simulink model "Combined"  (R2024b)
settings: Solver=VariableStepAuto  StartTime=0.0  StopTime=10.0  RelTol=1e-3
undefined symbols (not defined in the file): C_PFC, Co, Cr, D11, Delta, DiscIntNeverNeededParam, Fnom, Fr_I, fs_LCC_max, fs_LCC_min, Ki_LLC, Ki_V, Kp_I, Kp_LLC, Kp_V, Kr_I, L_PFC, Limit_V, Lm, Lr, Np, Ns, Po_nom, RL_PFC, Ts_Control, Ts_Power, Vnom_ac, Vo_nom, Vref_LCC_max, Vref_LCC_min
libraries: spsSeriesRLCBranchLib x9, spsCurrentMeasurementLib x7, spsDiodeLib x7, MyLibrary x6, spsVoltageMeasurementLib x5, spsMeanLib x4, spsOnDelayLib x3, slpidlib x2, spsPWMGeneratorDCDCLib x2, spsFourierLib x2, simulink x2, spspowerguiLib x2
settings Model: Creator=chang  LastModifiedBy=chang

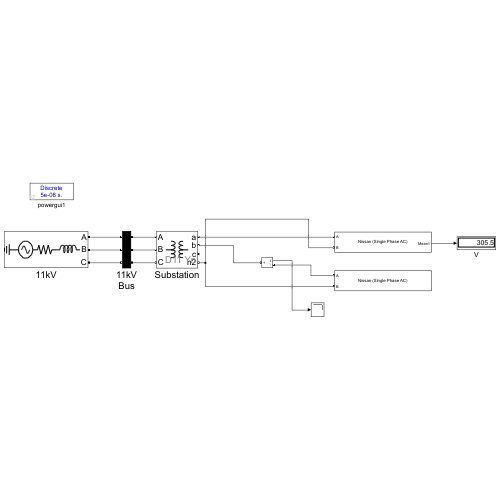
[thumbnail: Simulink's stored preview of the top-level diagram]
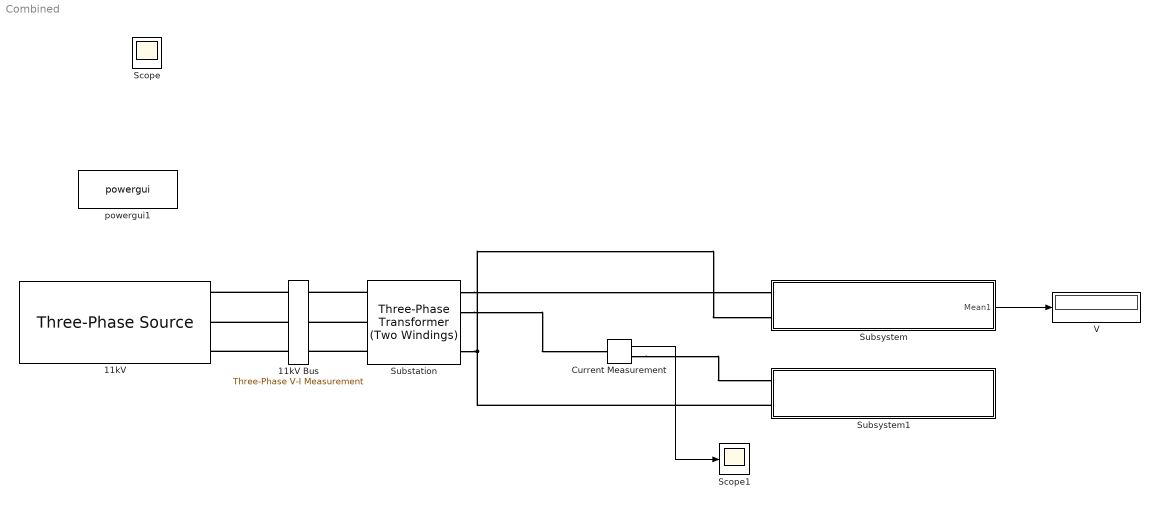
== system Combined ==
  11kV : spsThreePhaseSourceLib/Three-Phase Source  InternalConnection=Yg  VoltagePhases=off  Voltage=11e3  PhaseAngle=0  Voltage_phases=[25e3 25e3 25e3]/sqrt(3)  PhaseAngles_phases=[0 -120 +120]  Frequency=50  NonIdealSource=on  SpecifyImpedance=on  Resistance=0.8929  Inductance=16.58e-3  ShortCircuitLevel=15e6  BaseVoltage=11e3  XRratio=7  BusType=swing  Pref=10e3  Qref=0  Prefabc=[10e3, 10e3, 10e3]  Qrefabc=[0, 0, 0]  Qmin=-inf  Qmax=inf
  11kV Bus : spsThreePhaseVIMeasurementLib/Three-Phase V-I Measurement  VoltageMeasurement=no  SetLabelV=off  LabelV=Vabc  Vpu=off  VpuLL=off  CurrentMeasurement=no  SetLabelI=off  LabelI=Iabc  Ipu=off  Pbase=100e6  Vbase=500e3  OutputType=Complex  PhasorSimulation=off  PSBequivalent=0
  Current Measurement : spsCurrentMeasurementLib/Current Measurement  PhasorSimulation=off  OutputType=Complex  PSBequivalent=0
  Scope1 : Scope
  Substation : spsThreePhaseTransformerTwoWindingsLib/Three-Phase Transformer (Two Windings)  Winding1Connection=Delta (D11)  Winding2Connection=Yn  CoreType=Three single-phase transformers  SetSaturation=off  Hysteresis=off  DataFile='hysteresis'  SetInitialFlux=off  Measurements=None  UNITS=pu  NominalPower=[ 1e6 , 50 ]  Winding1=[11e3 0.0019999 0.080002]  Winding2=[0.4e3 0.002 0.08]  Rm=500.01  Lm=500  L0=0.5  Saturation=[0 0;0.0024 1.2;0.99999 1.52]  InitialFluxes=[ 0.8 , -0.8 , 0.7 ]  BreakLoop=off  DiscreteSolver=Trapezoidal iterative  DataType=off  TransfoNumber=1
  Subsystem : Subsystem
      mask Display: disp('Nissan (Single Phase AC)');
  Subsystem1 : Subsystem
      mask Display: disp('Nissan (Single Phase AC)');
  V : Display
  powergui1 : spspowerguiLib/powergui  Priority=1  SimulationMode=Discrete  SampleTime=Ts_Power  frequency=60  Iterations=50  frequencyindice=0  Pbase=100e6  ErrMax=1e-4  UnitsV=kV  UnitsW=MW  buscounter=0  FunctionMessages=off  echomessages=off  EnableUseOfTLC=off  CurrentSourceSwitches=off  DisableSnubberDevices=off  DisableRonSwitches=off  DisableVfSwitches=off  DisplayEquations=off  AutomaticDiscreteSolvers=off  SolverType=Tustin/Backward Euler (TBE)  Interpol=off  ExternalGateDelay=off  methode=off  Ts=100  x0status=blocks  SPID=on  SwTol=0  HookPort=off  NonlinearTolerance=1e-4  nMaxIteration=100  ContinueOnMaxIteration=off  RestoreLinks=warning  ResistiveCurrentMeasurement=off  Frange=[0:2:500]  Ylog=off  Xlog=on  ShowGrid=off  save=off  variable=ZData  structure=0  ZoomFFT=off  StartTime=0.0  cycles=1  DisplayStyle=1  fundamental=60  FreqAxis=off  MaxFrequency=1000  frequencyindicesteady=1  RmsSteady=1  display=off
  Scope : Scope
  wires:
  Subsystem/1(Mean1) -> V/1
  Current Measurement/1 -> Scope1/1
  connections:
  11kV Bus/LConn1 -- 11kV/RConn1
  11kV Bus/LConn2 -- 11kV/RConn2
  11kV Bus/LConn3 -- 11kV/RConn3
  Substation/LConn1 -- 11kV Bus/RConn1
  Substation/LConn2 -- 11kV Bus/RConn2
  Substation/LConn3 -- 11kV Bus/RConn3
  Substation/RConn4 -- Subsystem1/LConn2 -- Subsystem/LConn2
  Substation/RConn1 -- Subsystem/LConn1
  Current Measurement/RConn1 -- Subsystem1/LConn1
  Substation/RConn2 -- Current Measurement/LConn1

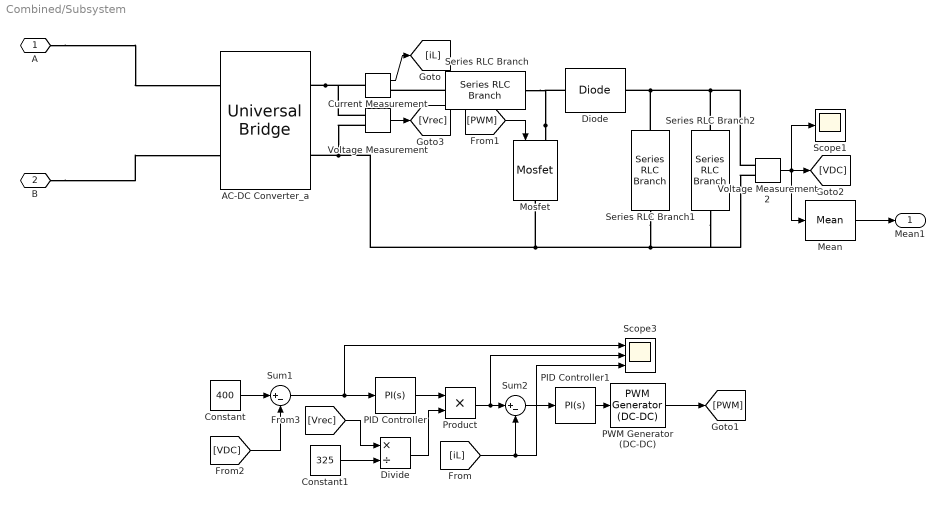
== system Combined/Subsystem ==
  AC-DC Converter_a : spsUniversalBridgeLib/Universal Bridge  Arms=2  SnubberResistance=1e5  SnubberCapacitance=inf  Device=Diodes  Ron=1e-3  Lon=0  ForwardVoltages="[  0  0  ]"  ForwardVoltage=0  GTOparameters=[ 10e-6 , 20e-6 ]  IGBTparameters=[ 1e-6 , 2e-6 ]  Measurements=None  Measurements_2=None  converterType=Rectifier
  Constant : Constant  Value=400
  Constant1 : Constant  Value=325
  Current Measurement : spsCurrentMeasurementLib/Current Measurement  PhasorSimulation=off  OutputType=Complex  PSBequivalent=0
  Diode : spsDiodeLib/Diode  Ron=0.001  Lon=0  Vf=0.8  IC=0  UseSnubber=0  Rs=inf  Cs=250e-9  Measurements=off
  Divide : Product  Inputs=*/
  Mean : spsMeanLib/Mean  Freq=100  Vinit=0  Ts=0
  Mosfet : spsMosfetLib/Mosfet  Ron=0.1  Lon=0  Rd=0.01  Vfd=0  IC=0  Rs=1e5  Cs=inf  Measurements=off
  PID Controller : slpidlib/PID Controller  Controller=PI  Form=Parallel  TimeDomain=Continuous-time  UseExternalTs=off  SampleTime=-1  IntegratorMethod=Forward Euler  FilterMethod=Forward Euler  ControllerParametersSource=internal  P=0.1  I=20  UseKiTs=off  D=0  UseExternalDerivativeSource=off  N=100  UseFilter=on  TunerSelectOption=Transfer Function Based (PID Tuner App)  InitialConditionSource=internal  InitialConditionForIntegrator=0  InitialConditionForFilter=0  DifferentiatorICPrevScaledInput=0  ExternalReset=none  TrackingMode=off  Kt=1  LimitOutput=off  SatLimitsSource=internal  UpperSaturationLimit=inf  LowerSaturationLimit=-inf  LinearizeAsGain=on  AntiWindupMode=none  Kb=1  LimitIntegrator=off  UpperIntegratorSaturationLimit=inf  LowerIntegratorSaturationLimit=-inf  POutMin=[]  POutMax=[]  IOutMin=[]  IOutMax=[]  DOutMin=[]  DOutMax=[]  NOutMin=[]  NOutMax=[]  SumOutMin=[]  SumOutMax=[]  SaturationOutMin=[]  SaturationOutMax=[]  PParamMin=[]  PParamMax=[]  IParamMin=[]  IParamMax=[]  DParamMin=[]  DParamMax=[]  NParamMin=[]  NParamMax=[]  KbParamMin=[]  KbParamMax=[]  KtParamMin=[]  KtParamMax=[]  KbOutMin=[]  KbOutMax=[]  KtOutMin=[]  KtOutMax=[]  IntegratorOutMin=[]  IntegratorOutMax=[]  FilterOutMin=[]  FilterOutMax=[]  SumI1OutMin=[]  SumI1OutMax=[]  SumI2OutMin=[]  SumI2OutMax=[]  SumI3OutMin=[]  SumI3OutMax=[]  SumI4OutMin=[]  SumI4OutMax=[]  SumDOutMin=[]  SumDOutMax=[]  DifferentiatorOutMin=[]  DifferentiatorOutMax=[]  FilterDiffOutCoefMin=[]  FilterDiffOutCoefMax=[]  ReciprocalOutMin=[]  ReciprocalOutMax=[]  SumDenOutMin=[]  SumDenOutMax=[]  SumNumOutMin=[]  SumNumOutMax=[]  DivideOutMin=[]  DivideOutMax=[]  UdiffTsProdOutMin=[]  UdiffTsProdOutMax=[]  NTsProdOutMin=[]  NTsProdOutMax=[]  UintegralTsProdOutMin=[]  UintegralTsProdOutMax=[]  UngainTsProdOutMin=[]  UngainTsProdOutMax=[]  ClampingZeroOutDataTypeStr=Inherit: Inherit via back propagation  ClampingZeroOutMin=[]  ClampingZeroOutMax=[]  FilterDenConstantOutDataTypeStr=Inherit: Inherit via back propagation  FilterDenConstantOutMin=[]  FilterDenConstantOutMax=[]  PCopyOutDataTypeStr=Inherit: Inherit via back propagation  PCopyOutMin=[]  PCopyOutMax=[]  NCopyOutDataTypeStr=Inherit: Inherit via back propagation  NCopyOutMin=[]  NCopyOutMax=[]  IntegratorContinuousStateAttributes=''  IntegratorStateMustResolveToSignalObject=off  IntegratorRTWStateStorageClass=Auto  FilterContinuousStateAttributes=''  FilterStateMustResolveToSignalObject=off  FilterRTWStateStorageClass=Auto  ParallelPVariant=InternalParameters  IdealPVariant=Disabled  IVariant=InternalParameters  DVariant=Disabled  IntegratorVariant=Continuous  SatVariant=Disabled  AWVariant=Passthrough  PCopyVariant=Disabled  TRVariant=Disabled  FdbkBlocksVariant=Forward  IdealPFdbkVariant=Disabled  SatFdbkVariant=Disabled  DerivativeFilterVariant=Disabled  NVariant=Disabled  NCopyVariant=Disabled_SignalSpec  FilterICVariant=Disabled  IntegratorICVariant=InternalICs  ExternalResetVariant=Disabled  TRSumVariant=Passthrough  SumFdbkVariant=Disabled  SumVariant=Sum_PI  TsampFilterVariant=InternalTs  TsampNgainVariant=Passthrough  TsampIntegralVariant=Disabled_SignalSpec  ExternalSaturationOutDataTypeStr=Inherit: Same as second input  DerivativeSourceVariant=Disabled  PreIntVariant=InternalPreInt
  PID Controller1 : slpidlib/PID Controller  Controller=PI  Form=Parallel  TimeDomain=Continuous-time  UseExternalTs=off  SampleTime=-1  IntegratorMethod=Forward Euler  FilterMethod=Forward Euler  ControllerParametersSource=internal  P=2000  I=0.25  UseKiTs=off  D=0  UseExternalDerivativeSource=off  N=100  UseFilter=on  TunerSelectOption=Transfer Function Based (PID Tuner App)  InitialConditionSource=internal  InitialConditionForIntegrator=0  InitialConditionForFilter=0  DifferentiatorICPrevScaledInput=0  ExternalReset=none  TrackingMode=off  Kt=1  LimitOutput=on  SatLimitsSource=internal  UpperSaturationLimit=1  LowerSaturationLimit=0  LinearizeAsGain=on  AntiWindupMode=none  Kb=1  LimitIntegrator=off  UpperIntegratorSaturationLimit=inf  LowerIntegratorSaturationLimit=-inf  POutMin=[]  POutMax=[]  IOutMin=[]  IOutMax=[]  DOutMin=[]  DOutMax=[]  NOutMin=[]  NOutMax=[]  SumOutMin=[]  SumOutMax=[]  SaturationOutMin=[]  SaturationOutMax=[]  PParamMin=[]  PParamMax=[]  IParamMin=[]  IParamMax=[]  DParamMin=[]  DParamMax=[]  NParamMin=[]  NParamMax=[]  KbParamMin=[]  KbParamMax=[]  KtParamMin=[]  KtParamMax=[]  KbOutMin=[]  KbOutMax=[]  KtOutMin=[]  KtOutMax=[]  IntegratorOutMin=[]  IntegratorOutMax=[]  FilterOutMin=[]  FilterOutMax=[]  SumI1OutMin=[]  SumI1OutMax=[]  SumI2OutMin=[]  SumI2OutMax=[]  SumI3OutMin=[]  SumI3OutMax=[]  SumI4OutMin=[]  SumI4OutMax=[]  SumDOutMin=[]  SumDOutMax=[]  DifferentiatorOutMin=[]  DifferentiatorOutMax=[]  FilterDiffOutCoefMin=[]  FilterDiffOutCoefMax=[]  ReciprocalOutMin=[]  ReciprocalOutMax=[]  SumDenOutMin=[]  SumDenOutMax=[]  SumNumOutMin=[]  SumNumOutMax=[]  DivideOutMin=[]  DivideOutMax=[]  UdiffTsProdOutMin=[]  UdiffTsProdOutMax=[]  NTsProdOutMin=[]  NTsProdOutMax=[]  UintegralTsProdOutMin=[]  UintegralTsProdOutMax=[]  UngainTsProdOutMin=[]  UngainTsProdOutMax=[]  ClampingZeroOutDataTypeStr=Inherit: Inherit via back propagation  ClampingZeroOutMin=[]  ClampingZeroOutMax=[]  FilterDenConstantOutDataTypeStr=Inherit: Inherit via back propagation  FilterDenConstantOutMin=[]  FilterDenConstantOutMax=[]  PCopyOutDataTypeStr=Inherit: Inherit via back propagation  PCopyOutMin=[]  PCopyOutMax=[]  NCopyOutDataTypeStr=Inherit: Inherit via back propagation  NCopyOutMin=[]  NCopyOutMax=[]  IntegratorContinuousStateAttributes=''  IntegratorStateMustResolveToSignalObject=off  IntegratorRTWStateStorageClass=Auto  FilterContinuousStateAttributes=''  FilterStateMustResolveToSignalObject=off  FilterRTWStateStorageClass=Auto  ParallelPVariant=InternalParameters  IdealPVariant=Disabled  IVariant=InternalParameters  DVariant=Disabled  IntegratorVariant=Continuous  SatVariant=Enabled  AWVariant=Passthrough  PCopyVariant=Disabled  TRVariant=Disabled  FdbkBlocksVariant=Forward  IdealPFdbkVariant=Disabled  SatFdbkVariant=Disabled  DerivativeFilterVariant=Disabled  NVariant=Disabled  NCopyVariant=Disabled_SignalSpec  FilterICVariant=Disabled  IntegratorICVariant=InternalICs  ExternalResetVariant=Disabled  TRSumVariant=Passthrough  SumFdbkVariant=Disabled  SumVariant=Sum_PI  TsampFilterVariant=InternalTs  TsampNgainVariant=Passthrough  TsampIntegralVariant=Disabled_SignalSpec  ExternalSaturationOutDataTypeStr=Inherit: Same as second input  DerivativeSourceVariant=Disabled  PreIntVariant=InternalPreInt
  PWM Generator (DC-DC) : spsPWMGeneratorDCDCLib/PWM Generator (DC-DC)  Fsw=50e3  Ts=1e-6
  Product : Product
  Scope1 : Scope
  Scope3 : Scope  NumInputPorts=3
  Series RLC Branch : spsSeriesRLCBranchLib/Series RLC Branch  LConnTagsString=__new0  RConnTagsString=__new0  BranchType=L  Resistance=1  Inductance=1e-3  SetiL0=off  InitialCurrent=0  Capacitance=1e-6  Setx0=off  InitialVoltage=0  Measurements=None
  Series RLC Branch1 : spsSeriesRLCBranchLib/Series RLC Branch  LConnTagsString=__new0  RConnTagsString=__new0  BranchType=C  Resistance=1  Inductance=1e-3  SetiL0=off  InitialCurrent=0  Capacitance=2000e-6  Setx0=off  InitialVoltage=0  Measurements=None
  Series RLC Branch2 : spsSeriesRLCBranchLib/Series RLC Branch  LConnTagsString=__new0  RConnTagsString=__new0  BranchType=R  Resistance=6.445  Inductance=1e-3  SetiL0=off  InitialCurrent=0  Capacitance=1e-6  Setx0=off  InitialVoltage=0  Measurements=Branch current
  Sum1 : Sum  Inputs=|+-
  Sum2 : Sum  Inputs=|+-
  Voltage Measurement : spsVoltageMeasurementLib/Voltage Measurement  PhasorSimulation=off  OutputType=Complex  PSBequivalent=0
  Voltage Measurement2 : spsVoltageMeasurementLib/Voltage Measurement  PhasorSimulation=off  OutputType=Complex  PSBequivalent=0
  A : PMIOPort  Side=Left
  B : PMIOPort  Port=2  Side=Left
  Mean1 : Outport
  wires:
  Sum1/1 -> Scope3/1, PID Controller/1
  Sum2/1 -> PID Controller1/1
  Voltage Measurement2/1 -> [VDC], Mean/1, Scope1/1
  Current Measurement/1 -> [iL]
  PID Controller1/1 -> PWM Generator (DC-DC)/1
  [Vrec] -> Divide/1
  [iL] -> Sum2/2, Scope3/3
  Mean/1 -> Mean1/1
  Product/1 -> Scope3/2, Sum2/1
  Divide/1 -> Product/2
  Voltage Measurement/1 -> [Vrec]
  PWM Generator (DC-DC)/1 -> [PWM]
  PID Controller/1 -> Product/1
  [PWM] -> Mosfet/1
  [VDC] -> Sum1/2
  Constant1/1 -> Divide/2
  Constant/1 -> Sum1/1
  connections:
  AC-DC Converter_a/RConn1 -- Voltage Measurement/LConn1 -- Current Measurement/LConn1
  Series RLC Branch1/RConn1 -- Voltage Measurement2/LConn2 -- Series RLC Branch2/RConn1 -- Voltage Measurement/LConn2 -- AC-DC Converter_a/RConn2 -- Mosfet/RConn1
  Series RLC Branch/LConn1 -- Current Measurement/RConn1
  B/RConn1 -- AC-DC Converter_a/LConn2
  Mosfet/LConn1 -- Diode/LConn1 -- Series RLC Branch/RConn1
  Series RLC Branch2/LConn1 -- Series RLC Branch1/LConn1 -- Diode/RConn1 -- Voltage Measurement2/LConn1
  A/RConn1 -- AC-DC Converter_a/LConn1

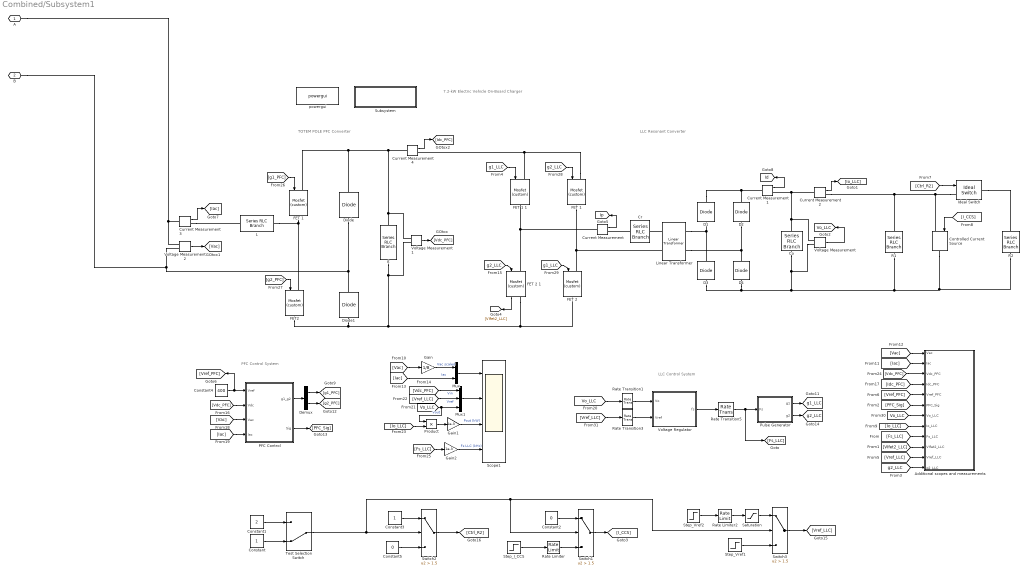
== system Combined/Subsystem1 ==
  note: TOTEM POLE PFC Converter
  note: 7.2-kW Electric Vehicle On-Board Charger
  note: LLC Control System
  note: PFC Control System
  note: LLC Resonant Converter
  Additional scopes and measurements : Subsystem
  C : spsSeriesRLCBranchLib/Series RLC Branch  LConnTagsString=__new0  RConnTagsString=__new0  BranchType=C  Resistance=1  Inductance=1e-3  SetiL0=off  InitialCurrent=0  Capacitance=C_PFC  Setx0=on  InitialVoltage=400  Measurements=None
  Co : spsSeriesRLCBranchLib/Series RLC Branch  LConnTagsString=__new0  RConnTagsString=__new0  BranchType=C  Resistance=1e-4  Inductance=200e-6  SetiL0=off  InitialCurrent=0  Capacitance=Co  Setx0=on  InitialVoltage=350  Measurements=None
  Constant : Constant
  Constant1 : Constant  Value=2
  Constant2 : Constant  Value=0
  Constant3 : Constant
  Constant4 : Constant  Value=400
  Constant5 : Constant  Value=0
  Controlled Current Source : spsControlledCurrentSourceLib/Controlled Current Source  Initialize=off  Source_Type=AC  Amplitude=0  Phase=0  Frequency=0  Measurements=None
  Cr : spsSeriesRLCBranchLib/Series RLC Branch  LConnTagsString=__new0  RConnTagsString=__new0  BranchType=C  Resistance=1e-4  Inductance=200e-6  SetiL0=off  InitialCurrent=0  Capacitance=Cr  Setx0=off  InitialVoltage=40  Measurements=None
  Current Measurement{,1..4} (5 alike) : spsCurrentMeasurementLib/Current Measurement  PhasorSimulation=off  OutputType=Complex  PSBequivalent=0
  D{1..4} (4 alike) : spsDiodeLib/Diode  Ron=Ron_Diode  Lon=0  Vf=Vf  IC=0  UseSnubber=off  Rs=1e6  Cs=inf  Measurements=off
  Demux : Demux  Outputs=2
  Diode : spsDiodeLib/Diode  Ron=Ron_Diode  Lon=0  Vf=Vf  IC=0  UseSnubber=0  Rs=1e6  Cs=inf  Measurements=off
  Diode1 : spsDiodeLib/Diode  Ron=Ron_Diode  Lon=0  Vf=Vf  IC=0  UseSnubber=0  Rs=1e6  Cs=inf  Measurements=off
  FET 1 : MyLibrary/Mosfet (custom)  Ron=Ron_FET  Lon=0  Rd=Ron_Diode  Vfd=Vf  IC=0  Rs=1e6  Cs=inf  Measurements=off
  "FET 1 " : MyLibrary/Mosfet (custom)  Ron=Ron_FET  Lon=0  Rd=Ron_Diode  Vfd=Vf  IC=0  Rs=1e6  Cs=inf  Measurements=off
  FET 1 1 : MyLibrary/Mosfet (custom)  Ron=Ron_FET  Lon=0  Rd=Ron_Diode  Vfd=Vf  IC=0  Rs=1e6  Cs=inf  Measurements=off
  "FET 2 " : MyLibrary/Mosfet (custom)  Ron=Ron_FET  Lon=0  Rd=Ron_Diode  Vfd=Vf  IC=0  Rs=1e6  Cs=inf  Measurements=off
  FET 2 1 : MyLibrary/Mosfet (custom)  Ron=Ron_FET  Lon=0  Rd=Ron_Diode  Vfd=Vf  IC=0  Rs=1e6  Cs=inf  Measurements=on
  FET2 : MyLibrary/Mosfet (custom)  Ron=Ron_FET  Lon=0  Rd=Ron_Diode  Vfd=Vf  IC=0  Rs=1e6  Cs=inf  Measurements=off
  Gain : Gain  Gain=1/8
  Gain1 : Gain  Gain=1e-3
  Gain2 : Gain  Gain=1e-3
  Ideal Switch : spsIdealSwitchLib/Ideal Switch  Ron=0.001  Lon=0  IC=0  Rs=1e6  Cs=inf  Measurements=off
  L : spsSeriesRLCBranchLib/Series RLC Branch  LConnTagsString=__new0  RConnTagsString=__new0  BranchType=RL  Resistance=RL_PFC  Inductance=L_PFC  SetiL0=off  InitialCurrent=0  Capacitance=1e-6  Setx0=off  InitialVoltage=0  Measurements=None
  Linear Transformer : spsLinearTransformerLib/Linear Transformer  UNITS=SI  NominalPower=[ 7000 100e3 ]  winding1="[Np   1e-2 Lr]"  winding2="[Ns  1e-2  1e-8 ]"  ThreeWindings=off  winding3=[3.15e+05 0.7938 0.084225]  RmLm=[1e4 Lm]  Measurements=None  DataType=on
  Mux : Mux  Inputs=2
  Mux1 : Mux  Inputs=3
  PFC Control : Subsystem
  Product : Product
  Pulse Generator : Subsystem
  R1 : spsSeriesRLCBranchLib/Series RLC Branch  LConnTagsString=__new0  RConnTagsString=__new0  BranchType=R  Resistance=Vo_nom^2/(0.01*Po_nom)  Inductance=200e-6  SetiL0=off  InitialCurrent=0  Capacitance=400e-6  Setx0=off  InitialVoltage=0  Measurements=None
  R2 : spsSeriesRLCBranchLib/Series RLC Branch  LConnTagsString=__new0  RConnTagsString=__new0  BranchType=R  Resistance=450^2/(Po_nom)  Inductance=200e-6  SetiL0=off  InitialCurrent=0  Capacitance=400e-6  Setx0=off  InitialVoltage=0  Measurements=None
  Rate Limiter : RateLimiter  RisingSlewLimit=200  FallingSlewLimit=-200  SampleTimeMode=inherited  InitialCondition=3
  Rate Limiter2 : RateLimiter  RisingSlewLimit=200*5  FallingSlewLimit=-200*5  SampleTimeMode=inherited  InitialCondition=250
  Rate Transition1 : RateTransition  OutPortSampleTime=Ts_Control
  Rate Transition3 : RateTransition  OutPortSampleTime=Ts_Control
  Rate Transition5 : RateTransition  InitialCondition=200e3  OutPortSampleTime=Ts_Power
  Saturation : Saturate  UpperLimit=Vref_LCC_max  LowerLimit=Vref_LCC_min
  Scope1 : Scope  NumInputPorts=4
  Step_I_CCS : Step  Time=0.2  Before=3  After=18  SampleTime=Ts_Power
  Step_Vref1 : Step  Time=0.1  Before=350  After=400  SampleTime=Ts_Power
  Step_Vref2 : Step  Time=0.1  Before=250  After=450  SampleTime=Ts_Power
  Subsystem : Subsystem
      settings: OpenFcn=edit('OBC_v1_data');
      mask Display: disp('Double-click to open\n parameters file');
  Switch1 : Switch  Criteria=u2 > Threshold  Threshold=1.5  SaturateOnIntegerOverflow=off  InputSameDT=off
  Switch2 : Switch  Criteria=u2 > Threshold  Threshold=1.5  SaturateOnIntegerOverflow=off  InputSameDT=off
  Switch3 : Switch  Criteria=u2 > Threshold  Threshold=1.5  SaturateOnIntegerOverflow=off  InputSameDT=off
  Test Selection Switch : ManualSwitch  CurrentSetting=0
  Voltage Measurement : spsVoltageMeasurementLib/Voltage Measurement  PhasorSimulation=off  OutputType=Complex  PSBequivalent=0
  Voltage Measurement1 : spsVoltageMeasurementLib/Voltage Measurement  PhasorSimulation=off  OutputType=Complex  PSBequivalent=0
  Voltage Measurement2 : spsVoltageMeasurementLib/Voltage Measurement  PhasorSimulation=off  OutputType=Complex  PSBequivalent=0
  Voltage Regulator : Subsystem
  powergui : spspowerguiLib/powergui  Priority=1  SimulationMode=Discrete  SampleTime=Ts_Power  frequency=60  Iterations=50  frequencyindice=0  Pbase=100e6  ErrMax=1e-4  UnitsV=kV  UnitsW=MW  buscounter=0  FunctionMessages=off  echomessages=off  EnableUseOfTLC=off  CurrentSourceSwitches=off  DisableSnubberDevices=off  DisableRonSwitches=off  DisableVfSwitches=off  DisplayEquations=off  AutomaticDiscreteSolvers=off  SolverType=Tustin/Backward Euler (TBE)  Interpol=off  ExternalGateDelay=off  methode=off  Ts=100  x0status=blocks  SPID=on  SwTol=0  HookPort=off  NonlinearTolerance=1e-4  nMaxIteration=100  ContinueOnMaxIteration=off  RestoreLinks=warning  ResistiveCurrentMeasurement=off  Frange=[0:2:500]  Ylog=off  Xlog=on  ShowGrid=off  save=off  variable=ZData  structure=0  ZoomFFT=off  StartTime=0.0  cycles=1  DisplayStyle=1  fundamental=60  FreqAxis=off  MaxFrequency=1000  frequencyindicesteady=1  RmsSteady=1  display=off
  A : PMIOPort  Side=Left
  B : PMIOPort  Port=2  Side=Left
  tag scope: Id=global, Ip=global, Vo_LLC=global, g1_LLC=global, g2_LLC=global
  wires:
  Rate Transition5/1 -> [Fs_LLC], Pulse Generator/1(Fs)
  Voltage Measurement2/1 -> [Vac]
  Rate Transition1/1 -> Voltage Regulator/1(Vo)
  Voltage Regulator/1(fs) -> Rate Transition5/1
  Rate Transition3/1 -> Voltage Regulator/2(Vref)
  [Vdc_PFC] -> PFC Control/2(Vdc)
  Constant3/1 -> Switch2/1
  Rate Limiter2/1 -> Saturation/1
  Mux/1 -> Scope1/1
  Gain2/1 -> Scope1/4  "Fs LLC (kHz)"
  [Vdc_PFC] -> Additional scopes and measurements/3(Vdc_PFC)
  [Vref_LLC] -> Additional scopes and measurements/11(Vref_LLC)
  [Io_LLC] -> Additional scopes and measurements/8(Io_LLC)
  [g2_LLC] -> Additional scopes and measurements/12(g2_LLC)
  [Vo_LLC] -> Product/1, Mux1/3  "Vout"
  [Fs_LLC] -> Gain2/1
  Current Measurement3/1 -> [Iac]
  [g2_LLC] -> "FET 1 "/1
  [Idc_PFC] -> Additional scopes and measurements/4(Idc_PFC)
  [Vo_LLC] -> Additional scopes and measurements/7(Vo_LLC)
  [g2_PFC] -> FET2/1
  [Vac] -> Gain/1
  [Vref_PFC] -> Additional scopes and measurements/5(Vref_PFC)
  Voltage Measurement1/1 -> [Vdc_PFC]
  Constant1/1 -> Test Selection Switch/1
  [Vo_LLC] -> Rate Transition1/1
  Constant2/1 -> Switch1/1
  Gain/1 -> Mux/1  "Vac scaled"
  [Iac] -> PFC Control/4(Iac)
  Saturation/1 -> Switch3/1
  Pulse Generator/2(g2) -> [g2_LLC]
  [Iac] -> Mux/2  "Iac"
  Step_I_CCS/1 -> Rate Limiter/1
  [Vdc_PFC] -> Mux1/1  "Vin"
  PFC Control/2(Sig) -> [PFC_Sig]
  Voltage Measurement/1 -> [Vo_LLC]
  Rate Limiter/1 -> Switch1/3
  PFC Control/1(g1_g2) -> Demux/1
  Switch3/1 -> [Vref_LLC]
  [Iac] -> Additional scopes and measurements/2(Iac)
  [g1_PFC] -> FET 1/1
  [g1_LLC] -> FET 1 1/1
  FET 2 1/1 -> [VIfet2_LLC]
  Demux/1 -> [g1_PFC]
  Current Measurement/1 -> [Ip]
  Pulse Generator/1(g1) -> [g1_LLC]
  Test Selection Switch/1 -> Switch3/2, Switch1/2, Switch2/2
  [Fs_LLC] -> Additional scopes and measurements/9(Fs_LLC)
  [g1_LLC] -> "FET 2 "/1
  [Vac] -> PFC Control/3(Vac)
  Demux/2 -> [g2_PFC]
  Switch1/1 -> [I_CCS]
  Mux1/1 -> Scope1/2
  Constant/1 -> Test Selection Switch/2
  [Vref_LLC] -> Rate Transition3/1
  Step_Vref2/1 -> Rate Limiter2/1
  [Io_LLC] -> Product/2
  Current Measurement1/1 -> [Id]
  Product/1 -> Gain1/1
  [Vref_LLC] -> Mux1/2  "Vref"
  Current Measurement2/1 -> [Io_LLC]
  Current Measurement4/1 -> [Idc_PFC]
  [I_CCS] -> Controlled Current Source/1
  Constant4/1 -> [Vref_PFC], PFC Control/1(Vref)
  [Vac] -> Additional scopes and measurements/1(Vac)
  [VIfet2_LLC] -> Additional scopes and measurements/10(VIfet2_LLC)
  Constant5/1 -> Switch2/3
  Gain1/1 -> Scope1/3  "Pout (kW)"
  Switch2/1 -> [Ctrl_R2]
  [Ctrl_R2] -> Ideal Switch/1
  Step_Vref1/1 -> Switch3/3
  [g2_LLC] -> FET 2 1/1
  [PFC_Sig] -> Additional scopes and measurements/6(PFC_Sig)
  connections:
  D4/RConn1 -- D2/LConn1 -- Linear Transformer/RConn2
  Ideal Switch/LConn1 -- Current Measurement2/RConn1 -- R1/LConn1 -- Controlled Current Source/LConn1
  Voltage Measurement2/LConn2 -- B/RConn1 -- Diode/LConn1 -- Diode1/RConn1
  Voltage Measurement/LConn2 -- Co/RConn1 -- D4/LConn1 -- D3/LConn1 -- R2/RConn1 -- Controlled Current Source/RConn1 -- R1/RConn1
  D1/RConn1 -- D2/RConn1 -- Current Measurement1/LConn1
  Current Measurement1/RConn1 -- Current Measurement2/LConn1 -- Voltage Measurement/LConn1 -- Co/LConn1
  C/LConn1 -- Current Measurement4/LConn1 -- Diode/RConn1 -- FET 1/LConn1 -- Voltage Measurement1/LConn1
  FET 1 1/RConn1 -- FET 2 1/LConn1 -- Current Measurement/LConn1
  "FET 1 "/LConn1 -- FET 1 1/LConn1 -- Current Measurement4/RConn1
  Voltage Measurement2/LConn1 -- A/RConn1 -- Current Measurement3/LConn1
  "FET 2 "/RConn1 -- C/RConn1 -- Voltage Measurement1/LConn2 -- FET2/RConn1 -- Diode1/LConn1 -- FET 2 1/RConn1
  D3/RConn1 -- D1/LConn1 -- Linear Transformer/RConn1
  FET2/LConn1 -- L/RConn1 -- FET 1/RConn1
  "FET 1 "/RConn1 -- Linear Transformer/LConn2 -- "FET 2 "/LConn1
  Ideal Switch/RConn1 -- R2/LConn1
  Linear Transformer/LConn1 -- Cr/RConn1
  Current Measurement3/RConn1 -- L/LConn1
  Cr/LConn1 -- Current Measurement/RConn1

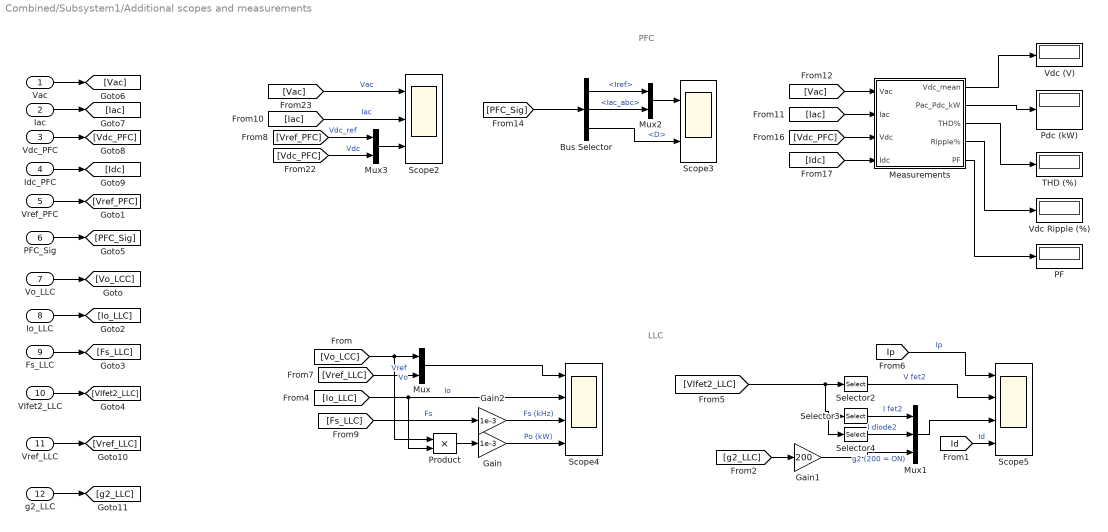
== system Combined/Subsystem1/Additional scopes and measurements ==
  note: PFC
  note: LLC
  Vac : Inport
  Iac : Inport  Port=2
  Vdc_PFC : Inport  Port=3
  Idc_PFC : Inport  Port=4
  Vref_PFC : Inport  Port=5
  PFC_Sig : Inport  Port=6
  Vo_LLC : Inport  Port=7
  Io_LLC : Inport  Port=8
  Fs_LLC : Inport  Port=9
  VIfet2_LLC : Inport  Port=10
  Vref_LLC : Inport  Port=11
  g2_LLC : Inport  Port=12
  Bus Selector : BusSelector  OutputSignals=Iref,Iac_abc,D
  Gain : Gain  Gain=1e-3
  Gain1 : Gain  Gain=200
  Gain2 : Gain  Gain=1e-3
  "Measurements " : Subsystem
  Mux : Mux  Inputs=2
  Mux1 : Mux  Inputs=3
  Mux2 : Mux  Inputs=2
  Mux3 : Mux  Inputs=2
  PF : Display
      settings: Format=bank  Decimation=100
  "Pdc (kW) " : Display
      settings: Format=bank  Decimation=100
  Product : Product
  Scope2 : Scope  NumInputPorts=3
  Scope3 : Scope  NumInputPorts=2
  Scope4 : Scope  NumInputPorts=4
  Scope5 : Scope  NumInputPorts=4
  Selector2 : Selector  InputPortWidth=3  IndexOptions=Index vector (dialog)  Indices=2  OutputSizes=1
  Selector3 : Selector  InputPortWidth=3  IndexOptions=Index vector (dialog)  Indices=1  OutputSizes=1
  Selector4 : Selector  InputPortWidth=3  IndexOptions=Index vector (dialog)  Indices=3  OutputSizes=1
  "THD (%) " : Display
      settings: Format=bank  Decimation=100
  "Vdc (V) " : Display
      settings: Format=bank  Decimation=100
  Vdc Ripple (%) : Display
      settings: Format=bank  Decimation=100
  wires:
  Mux/1 -> Scope4/1
  [VIfet2_LLC] -> Selector4/1, Selector3/1, Selector2/1
  Selector2/1 -> Scope5/2  "V fet2"
  [Vac] -> Scope2/1  "Vac"
  Gain/1 -> Scope4/4  "Po (kW)"
  Mux1/1 -> Scope5/3
  [Ip] -> Scope5/1  "Ip"
  Selector4/1 -> Mux1/2  "I diode2"
  Bus Selector/3 -> Scope3/2  "<D>"
  Bus Selector/1 -> Mux2/1  "<Iref>"
  Bus Selector/2 -> Mux2/2  "<Iac_abc>"
  [Vo_LCC] -> Product/1, Mux/1  "Vo"
  [Vref_LLC] -> Mux/2  "Vref"
  Selector3/1 -> Mux1/1  "I fet2"
  "Measurements "/2(Pac_Pdc_kW) -> "Pdc (kW) "/1
  "Measurements "/4(Ripple%) -> Vdc Ripple (%)/1
  [Vdc_PFC] -> "Measurements "/3(Vdc)
  [Io_LLC] -> Product/2, Scope4/2  "Io"
  Mux2/1 -> Scope3/1
  Product/1 -> Gain/1
  [Vdc_PFC] -> Mux3/2  "Vdc"
  Mux3/1 -> Scope2/3
  [Id] -> Scope5/4  "Id"
  [PFC_Sig] -> Bus Selector/1
  [Idc] -> "Measurements "/4(Idc)
  [Vref_PFC] -> Mux3/1  "Vdc_ref"
  "Measurements "/5(PF) -> PF/1
  [Fs_LLC] -> Gain2/1  "Fs"
  "Measurements "/1(Vdc_mean) -> "Vdc (V) "/1
  [Iac] -> Scope2/2  "Iac"
  [Vac] -> "Measurements "/1(Vac)
  "Measurements "/3(THD%) -> "THD (%) "/1
  [Iac] -> "Measurements "/2(Iac)
  Vo_LLC/1 -> [Vo_LCC]
  Io_LLC/1 -> [Io_LLC]
  Fs_LLC/1 -> [Fs_LLC]
  VIfet2_LLC/1 -> [VIfet2_LLC]
  Vac/1 -> [Vac]
  Iac/1 -> [Iac]
  Vdc_PFC/1 -> [Vdc_PFC]
  Idc_PFC/1 -> [Idc]
  Vref_PFC/1 -> [Vref_PFC]
  PFC_Sig/1 -> [PFC_Sig]
  Vref_LLC/1 -> [Vref_LLC]
  g2_LLC/1 -> [g2_LLC]
  [g2_LLC] -> Gain1/1
  Gain1/1 -> Mux1/3  "g2 (200 = ON)"
  Gain2/1 -> Scope4/3  "Fs (kHz)"

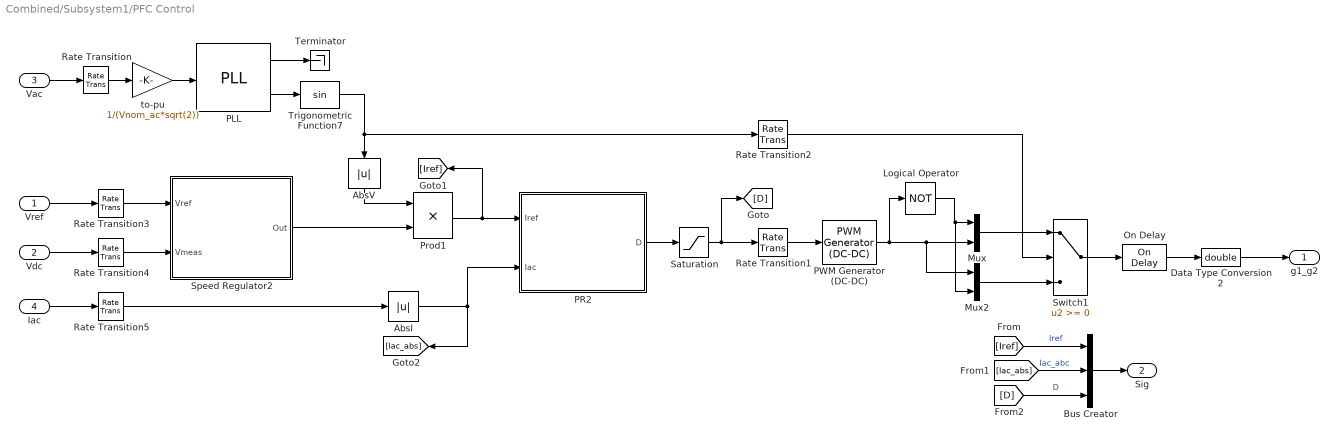
== system Combined/Subsystem1/PFC Control ==
  Vref : Inport
  Vdc : Inport  Port=2
  Vac : Inport  Port=3
  Iac : Inport  Port=4
  AbsI : Abs  SaturateOnIntegerOverflow=off
  AbsV : Abs  SaturateOnIntegerOverflow=off
  Bus Creator : BusCreator  Inputs=3
  Data Type Conversion2 : DataTypeConversion  OutDataTypeStr=double  SaturateOnIntegerOverflow=off  RndMeth=Floor
  Logical Operator : Logic  Operator=NOT  AllPortsSameDT=off  OutDataTypeStr=float('double')
  Mux : Mux  Inputs=2
  Mux2 : Mux  Inputs=2
  On Delay : spsOnDelayLib/On Delay  DelayType=On delay  delay=DT_PFC  ic=0  Ts=Ts_Power
  PLL : spsPLLLib/PLL  Fmin=0.9*Fnom  Par_Init=[0, Fnom]  ParK=[180, 3200, 1]  TcD=1e-4  MaxRateChangeFreq=12  FilterCutOffFreq=25  Ts=Ts_Control  AGC=on
  PR2 : Subsystem  mask(Current Regulator (Pr)){Kp=Kp_I, Kr=Kr_I, Fr=Fr_I}
      mask prompts: Kp "Proportional gain"; Kr "Resonant gain"; Fr "Resonant frequency (Hz)"
      mask help: This block implements a currentregulator using a PR controller.
      mask Display: disp('Current Regulator\n PR');
  PWM Generator (DC-DC) : spsPWMGeneratorDCDCLib/PWM Generator (DC-DC)  Fsw=Fsw  Ts=Ts_Power
  Prod1 : Product
  Rate Transition{,3..5} (4 alike) : RateTransition  OutPortSampleTime=Ts_Control
  Rate Transition1 : RateTransition  OutPortSampleTime=Ts_Power
  Rate Transition2 : RateTransition  OutPortSampleTime=Ts_Power
  Saturation : Saturate  UpperLimit=1  LowerLimit=0
  Speed Regulator2 : Subsystem  DialogController=POWERSYS.PowerSysDialog  mask(Voltage Regulator){Kp=Kp_V, Ki=Ki_V, Limit_wreg=Limit_V, Init=0, Ts=Ts_Control}
      mask prompts: Kp "Proportional gain (Kp):"; Ki "Integral gain (Ki):"; Limit_wreg "Output limits"; Init "Output initial value:"; Ts "Sample time:"
      mask help: This block implements a voltage regulator using an ant-windup PI controller.
      mask Display: disp('Voltage\nRegulator');
  Switch1 : Switch  SaturateOnIntegerOverflow=off  InputSameDT=off
  Terminator : Terminator
  Trigonometric Function7 : Trigonometry
  to-pu : Gain  Gain=1/(Vnom_ac*sqrt(2))
  g1_g2 : Outport  PortDimensions=2
  Sig : Outport  Port=2
  wires:
  Vdc/1 -> Rate Transition4/1
  Speed Regulator2/1(Out) -> Prod1/2
  Vac/1 -> Rate Transition/1
  AbsV/1 -> Prod1/1
  Vref/1 -> Rate Transition3/1
  Prod1/1 -> PR2/1(Iref), [Iref]
  AbsI/1 -> PR2/2(Iac), [Iac_abs]
  Saturation/1 -> [D], Rate Transition1/1
  Mux/1 -> Switch1/1
  Mux2/1 -> Switch1/3
  Rate Transition1/1 -> PWM Generator (DC-DC)/1
  Bus Creator/1 -> Sig/1
  [Iref] -> Bus Creator/1  "Iref"
  [Iac_abs] -> Bus Creator/2  "Iac_abc"
  [D] -> Bus Creator/3  "D"
  Switch1/1 -> On Delay/1
  PWM Generator (DC-DC)/1 -> Logical Operator/1, Mux2/1, Mux/2
  to-pu/1 -> PLL/1
  PLL/2 -> Trigonometric Function7/1
  Trigonometric Function7/1 -> AbsV/1, Rate Transition2/1
  PLL/1 -> Terminator/1
  PR2/1(D) -> Saturation/1
  Logical Operator/1 -> Mux2/2, Mux/1
  Rate Transition2/1 -> Switch1/2
  Rate Transition/1 -> to-pu/1
  Rate Transition3/1 -> Speed Regulator2/1(Vref)
  Rate Transition4/1 -> Speed Regulator2/2(Vmeas)
  Rate Transition5/1 -> AbsI/1
  Iac/1 -> Rate Transition5/1
  On Delay/1 -> Data Type Conversion2/1
  Data Type Conversion2/1 -> g1_g2/1

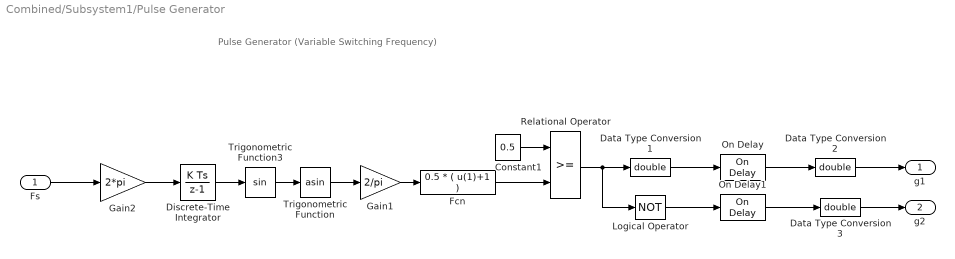
== system Combined/Subsystem1/Pulse Generator ==
  note: Pulse Generator
      | (Variable Switching Frequency)
  Fs : Inport
  Constant1 : Constant  Value=0.5
  Data Type Conversion1 : DataTypeConversion  OutDataTypeStr=double  SaturateOnIntegerOverflow=off  RndMeth=Floor
  Data Type Conversion2 : DataTypeConversion  OutDataTypeStr=double  SaturateOnIntegerOverflow=off  RndMeth=Floor
  Data Type Conversion3 : DataTypeConversion  OutDataTypeStr=double  SaturateOnIntegerOverflow=off  RndMeth=Floor
  Discrete-Time Integrator : DiscreteIntegrator  SampleTime=Ts_Power  ICPrevOutput=DiscIntNeverNeededParam  ICPrevScaledInput=DiscIntNeverNeededParam
  Fcn : Fcn  Expr=0.5 * ( u(1)+1 )
  Gain1 : Gain  Gain=2/pi  SaturateOnIntegerOverflow=on  OutDataTypeStr=Inherit: Same as input  ParamDataTypeStr=Inherit: Same as input
  Gain2 : Gain  Gain=2*pi  SaturateOnIntegerOverflow=on  OutDataTypeStr=Inherit: Same as input  ParamDataTypeStr=Inherit: Same as input
  Logical Operator : Logic  Operator=NOT  AllPortsSameDT=off  OutDataTypeStr=float('double')
  On Delay : spsOnDelayLib/On Delay  DelayType=On delay  delay=DT_LLC  ic=0  Ts=Ts_Power
  On Delay1 : spsOnDelayLib/On Delay  DelayType=On delay  delay=DT_LLC  ic=0  Ts=Ts_Power
  Relational Operator : RelationalOperator  OutDataTypeStr=boolean  InputSameDT=off
  Trigonometric Function : Trigonometry  Operator=asin
  Trigonometric Function3 : Trigonometry
  g1 : Outport  VectorParamsAs1DForOutWhenUnconnected=off
  g2 : Outport  Port=2  VectorParamsAs1DForOutWhenUnconnected=off
  wires:
  On Delay1/1 -> Data Type Conversion3/1
  On Delay/1 -> Data Type Conversion2/1
  Fs/1 -> Gain2/1
  Gain2/1 -> Discrete-Time Integrator/1
  Data Type Conversion1/1 -> On Delay/1
  Logical Operator/1 -> On Delay1/1
  Fcn/1 -> Relational Operator/2
  Relational Operator/1 -> Logical Operator/1, Data Type Conversion1/1
  Constant1/1 -> Relational Operator/1
  Discrete-Time Integrator/1 -> Trigonometric Function3/1
  Trigonometric Function/1 -> Gain1/1
  Gain1/1 -> Fcn/1
  Trigonometric Function3/1 -> Trigonometric Function/1
  Data Type Conversion2/1 -> g1/1
  Data Type Conversion3/1 -> g2/1

== system Combined/Subsystem1/Subsystem ==

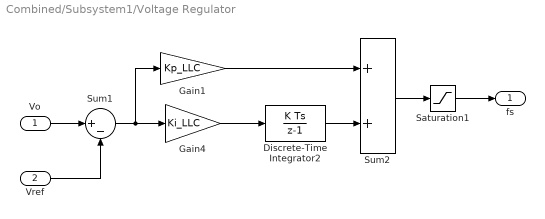
== system Combined/Subsystem1/Voltage Regulator ==
  Vo : Inport
  Vref : Inport  Port=2
  Discrete-Time Integrator2 : DiscreteIntegrator  InitialCondition=fs_LCC_min  SampleTime=Ts_Control  LimitOutput=on  UpperSaturationLimit=fs_LCC_max  LowerSaturationLimit=fs_LCC_min  ICPrevOutput=DiscIntNeverNeededParam  ICPrevScaledInput=DiscIntNeverNeededParam
  Gain1 : Gain  Gain=Kp_LLC  SaturateOnIntegerOverflow=on  OutDataTypeStr=Inherit: Same as input  ParamDataTypeStr=Inherit: Same as input
  Gain4 : Gain  Gain=Ki_LLC  SaturateOnIntegerOverflow=on  OutDataTypeStr=Inherit: Same as input  ParamDataTypeStr=Inherit: Same as input
  Saturation1 : Saturate  UpperLimit=fs_LCC_max  LowerLimit=fs_LCC_min
  Sum1 : Sum  Inputs=|+-  InputSameDT=on  SaturateOnIntegerOverflow=on  OutDataTypeStr=Inherit: Same as first input
  Sum2 : Sum  InputSameDT=on  SaturateOnIntegerOverflow=on  OutDataTypeStr=Inherit: Same as first input
  fs : Outport  VectorParamsAs1DForOutWhenUnconnected=off
  wires:
  Saturation1/1 -> fs/1
  Gain1/1 -> Sum2/1
  Sum2/1 -> Saturation1/1
  Discrete-Time Integrator2/1 -> Sum2/2
  Gain4/1 -> Discrete-Time Integrator2/1
  Sum1/1 -> Gain4/1, Gain1/1
  Vo/1 -> Sum1/1
  Vref/1 -> Sum1/2

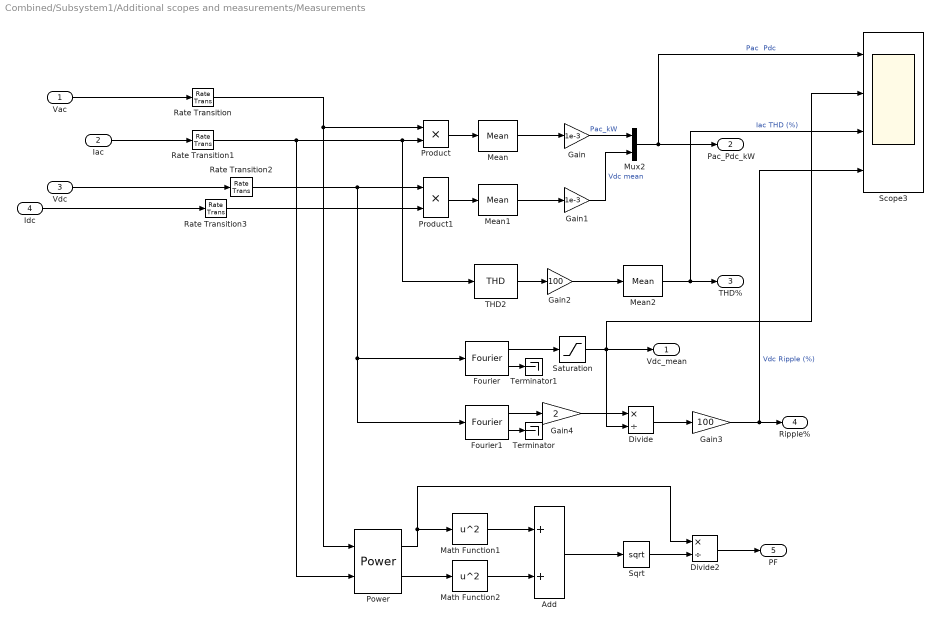
== system Combined/Subsystem1/Additional scopes and measurements/Measurements  ==
  Vac : Inport
  Iac : Inport  Port=2
  Vdc : Inport  Port=3
  Idc : Inport  Port=4
  Add : Sum
  Divide : Product  Inputs=*/
  Divide2 : Product  Inputs=*/
  Fourier : spsFourierLib/Fourier  Freq=Fnom  n=0  InInit=[0, 0]  Ts=Ts_Control
  Fourier1 : spsFourierLib/Fourier  Freq=Fnom  n=2  InInit=[0, 0]  Ts=Ts_Control
  Gain : Gain  Gain=1e-3
  Gain1 : Gain  Gain=1e-3
  Gain2 : Gain  Gain=100
  Gain3 : Gain  Gain=100
  Gain4 : Gain  Gain=2
  Math Function1 : Math  Operator=square
  Math Function2 : Math  Operator=square
  Mean : spsMeanLib/Mean  Freq=Fnom  Vinit=0  Ts=Ts_Control
  Mean1 : spsMeanLib/Mean  Freq=Fnom  Vinit=0  Ts=Ts_Control
  Mean2 : spsMeanLib/Mean  Freq=Fnom  Vinit=0  Ts=Ts_Control
  Mux2 : Mux  Inputs=2
  Power : spsPowerLib/Power  Freq=Fnom  Vinit=[1, 0]  Iinit=[1, 0]  Ts=Ts_Control
  Product : Product
  Product1 : Product
  Rate Transition{,1..3} (4 alike) : RateTransition  OutPortSampleTime=Ts_Control
  Saturation : Saturate  UpperLimit=inf  LowerLimit=eps
  Scope3 : Scope  NumInputPorts=4
  Sqrt : Sqrt
  THD2 : spsTHDLib/THD  Freq=Fnom  Ts=Ts_Control
  Terminator : Terminator
  Terminator1 : Terminator
  Vdc_mean : Outport
  Pac_Pdc_kW : Outport  Port=2
  THD% : Outport  Port=3
  Ripple% : Outport  Port=4
  PF : Outport  Port=5
  wires:
  Gain1/1 -> Mux2/2  "Vdc mean"
  Product1/1 -> Mean1/1
  Mean/1 -> Gain/1
  Product/1 -> Mean/1
  Gain/1 -> Mux2/1  "Pac_kW"
  THD2/1 -> Gain2/1
  Mean1/1 -> Gain1/1
  Iac/1 -> Rate Transition1/1
  Mux2/1 -> Scope3/1, Pac_Pdc_kW/1  "Pac  Pdc"
  Gain2/1 -> Mean2/1
  Mean2/1 -> Scope3/3, THD%/1  "Iac THD (%)"
  Fourier/2 -> Terminator1/1
  Fourier/1 -> Saturation/1
  Saturation/1 -> Scope3/2, Vdc_mean/1, Divide/2
  Divide/1 -> Gain3/1
  Fourier1/1 -> Gain4/1
  Gain4/1 -> Divide/1
  Fourier1/2 -> Terminator/1
  Gain3/1 -> Scope3/4, Ripple%/1  "Vdc Ripple (%)"
  Power/1 -> Math Function1/1, Divide2/1
  Power/2 -> Math Function2/1
  Math Function1/1 -> Add/1
  Math Function2/1 -> Add/2
  Add/1 -> Sqrt/1
  Sqrt/1 -> Divide2/2
  Divide2/1 -> PF/1
  Rate Transition1/1 -> Power/2, THD2/1, Product/2
  Vdc/1 -> Rate Transition2/1
  Idc/1 -> Rate Transition3/1
  Rate Transition/1 -> Power/1, Product/1
  Vac/1 -> Rate Transition/1
  Rate Transition2/1 -> Product1/1, Fourier/1, Fourier1/1
  Rate Transition3/1 -> Product1/2

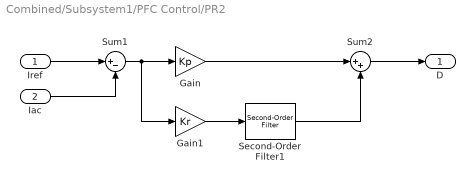
== system Combined/Subsystem1/PFC Control/PR2 ==
  Iref : Inport
  Iac : Inport  Port=2
  Gain : Gain  Gain=Kp
  Gain1 : Gain  Gain=Kr
  Second-Order Filter1 : spsSecondOrderFilterLib/Second-Order Filter  FilterType=Bandpass  Fo=Fr  Zeta=Zeta_I  Ts=Ts_Control  Initialize=off  Vac_Init="[0,  0,  60]"  Vdc_Init=0  PlotResponse=off  FreqRange=[0, 1000, 0.2]
  Sum1 : Sum  Inputs=|+-
  Sum2 : Sum  Inputs=|++
  D : Outport
  wires:
  Gain1/1 -> Second-Order Filter1/1
  Sum2/1 -> D/1
  Gain/1 -> Sum2/1
  Iac/1 -> Sum1/2
  Iref/1 -> Sum1/1
  Sum1/1 -> Gain1/1, Gain/1
  Second-Order Filter1/1 -> Sum2/2

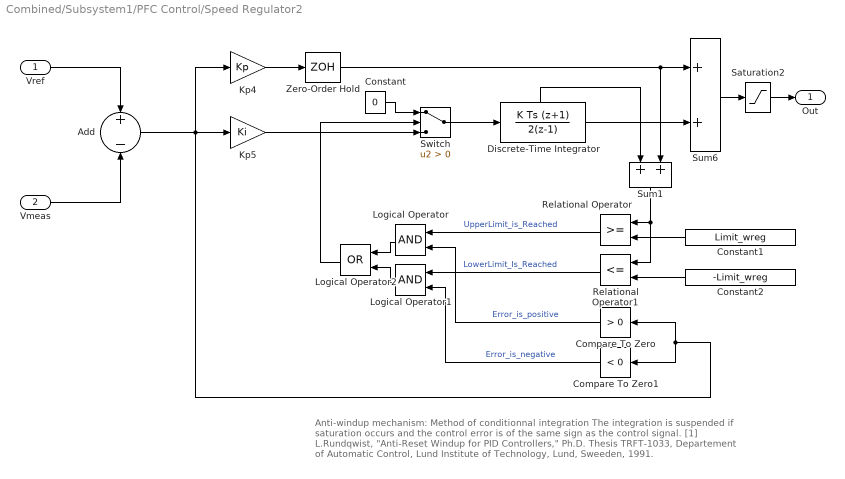
== system Combined/Subsystem1/PFC Control/Speed Regulator2 ==
  note: Anti-windup mechanism: Method of conditionnal integration
      |
      | The integration is suspended if saturation occurs and the
      | control error is of the same sign as the control signal.
      |
      | [1] L.Rundqwist, "Anti-Reset Windup for PID Controllers," Ph.D. Thesis TRFT-1033,
      | Departement of Automatic Control, Lund Institute of Technology, Lund, Sweeden, 1991.
  Vref : Inport  PortDimensions=1
  Vmeas : Inport  Port=2  PortDimensions=1
  Add : Sum  Inputs=+|-
  Compare To Zero : simulink/Logic and Bit Operations/Compare To Zero  relop=>  OutDataTypeStr=uint8  ZeroCross=off
  Compare To Zero1 : simulink/Logic and Bit Operations/Compare To Zero  relop=<  OutDataTypeStr=uint8  ZeroCross=off
  Constant : Constant  Value=0
  Constant1 : Constant  Value=Limit_wreg
  Constant2 : Constant  Value=-Limit_wreg
  Discrete-Time Integrator : DiscreteIntegrator  IntegratorMethod=Integration: Trapezoidal  InitialCondition=Init  SampleTime=Ts  LimitOutput=on  UpperSaturationLimit=Limit_wreg  LowerSaturationLimit=-Limit_wreg  ShowStatePort=on  ICPrevOutput=DiscIntNeverNeededParam  ICPrevScaledInput=DiscIntNeverNeededParam
  Kp4 : Gain  Gain=Kp  SaturateOnIntegerOverflow=on  SampleTime=Ts  OutDataTypeStr=Inherit: Same as input  ParamDataTypeStr=Inherit: Same as input
  Kp5 : Gain  Gain=Ki  SaturateOnIntegerOverflow=on  SampleTime=Ts  OutDataTypeStr=Inherit: Same as input  ParamDataTypeStr=Inherit: Same as input
  Logical Operator : Logic  AllPortsSameDT=off  OutDataTypeStr=boolean
  Logical Operator1 : Logic  AllPortsSameDT=off  OutDataTypeStr=boolean
  Logical Operator2 : Logic  Operator=OR  AllPortsSameDT=off  OutDataTypeStr=boolean
  Relational Operator : RelationalOperator  OutDataTypeStr=boolean  InputSameDT=off
  Relational Operator1 : RelationalOperator  Operator=<=  OutDataTypeStr=boolean  InputSameDT=off
  Saturation2 : Saturate  UpperLimit=Limit_wreg  LowerLimit=-Limit_wreg  SampleTime=Ts
  Sum1 : Sum  InputSameDT=on  SaturateOnIntegerOverflow=on  SampleTime=Ts  OutDataTypeStr=Inherit: Same as first input
  Sum6 : Sum  InputSameDT=on  SaturateOnIntegerOverflow=on  SampleTime=Ts  OutDataTypeStr=Inherit: Same as first input
  Switch : Switch  Criteria=u2 > Threshold  SaturateOnIntegerOverflow=off  InputSameDT=off
  Zero-Order Hold : ZeroOrderHold  SampleTime=Ts
  Out : Outport  SampleTime=Ts  InitialOutput=0  VectorParamsAs1DForOutWhenUnconnected=off
  wires:
  Kp5/1 -> Switch/3
  Switch/1 -> Discrete-Time Integrator/1
  Saturation2/1 -> Out/1
  Discrete-Time Integrator/1 -> Sum6/2
  Kp4/1 -> Zero-Order Hold/1
  Sum6/1 -> Saturation2/1
  Add/1 -> Compare To Zero/1, Compare To Zero1/1, Kp5/1, Kp4/1
  Compare To Zero1/1 -> Logical Operator1/2  "Error_is_negative"
  Logical Operator1/1 -> Logical Operator2/2
  Logical Operator/1 -> Logical Operator2/1
  Compare To Zero/1 -> Logical Operator/2  "Error_is_positive"
  Constant2/1 -> Relational Operator1/2
  Constant1/1 -> Relational Operator/2
  Relational Operator1/1 -> Logical Operator1/1  "LowerLimit_Is_Reached"
  Relational Operator/1 -> Logical Operator/1  "UpperLimit_is_Reached"
  Logical Operator2/1 -> Switch/2
  Sum1/1 -> Relational Operator/1, Relational Operator1/1
  Discrete-Time Integrator/State -> Sum1/1
  Zero-Order Hold/1 -> Sum6/1, Sum1/2
  Constant/1 -> Switch/1
  Vref/1 -> Add/1
  Vmeas/1 -> Add/2
